simulink model "bpsk_simulink"  (Simulink 7.3)
settings: Solver=ode45  StartTime=0.0  StopTime=10.0  RelTol=1e-3
undefined symbols (not defined in the file or in its folder): get
libraries: commsink2 x4, commdigbbndpm3 x2, commfilt2 x2, dspsrcs4 x2, commchan3 x1, commrandsrc2 x1, commphrec2 x1, commrflib2 x1
settings Model: Creator=joneskoo  LastModifiedBy=joneskoo

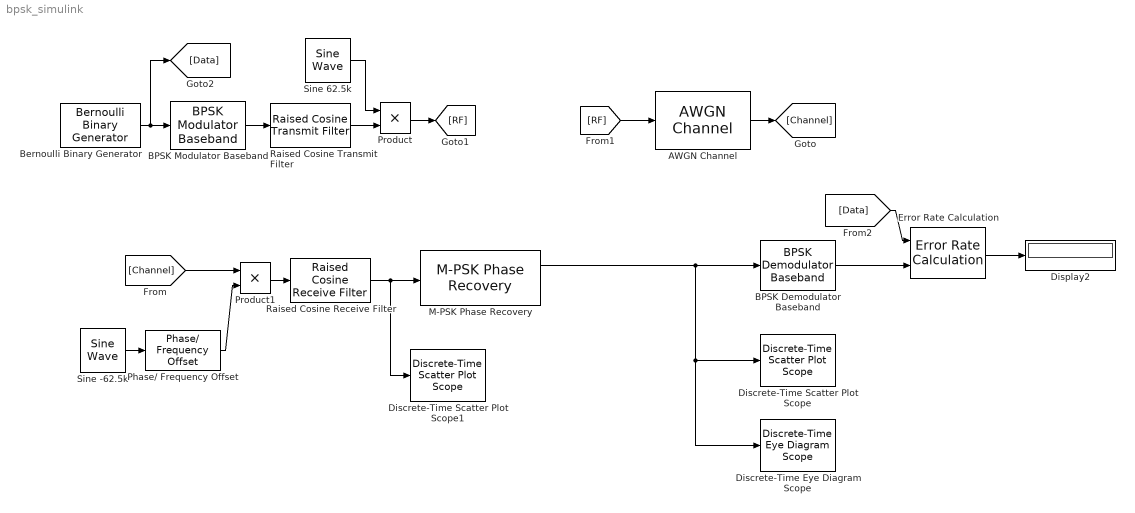
== system bpsk_simulink ==
  AWGN Channel : commchan3/AWGN Channel  SystemSampleTime=-1  seed=67  noiseMode="Signal to noise ratio  (SNR)"  EbNodB=40  EsNodB=10  SNRdB=15  bitsPerSym=1  Ps=1  Tsym=1  variance=1
  BPSK Demodulator Baseband : commdigbbndpm3/BPSK Demodulator Baseband  DialogController=commDDGCreate  DialogControllerArgs=DataTag0  Ph=0  DecType=Hard decision  VarSource=Dialog  Variance=1  outDtype=Inherit via internal rule  derotateFactorWordLen=16
  BPSK Modulator Baseband : commdigbbndpm3/BPSK Modulator Baseband  DialogController=commDDGCreate  DialogControllerArgs=DataTag1  SystemSampleTime=-1  Ph=0  outDtype=double  outWordLen=16  outUDDataType=sfix(16)  outFracLenMode=Best precision  outFracLen=15
  Bernoulli Binary Generator : commrandsrc2/Bernoulli Binary Generator  DialogController=commDDGCreate  DialogControllerArgs=DataTag2  SystemSampleTime=-1  P=0.5  seed=61  Ts=64/500000  frameBased=off  sampPerFrame=4  orient=off  outDataType=double
  Discrete-Time Eye Diagram Scope : commsink2/Discrete-Time Eye Diagram Scope  Tag=EyeDiagram  SystemSampleTime=-1  sampPerSymb=64  offsetEye=0  symbPerTrace=1  numTraces=40  numNewFrames=10  LineStyles=-  LineColors=b  dupPoints=on  fading=on  render=on  AxisGrid=on  yMin=-3.15  yMax=3.15  inphaseLabel=In-phase Amplitude  quadratureLabel=Quadrature Amplitude  openScopeAtSimStart=on  dispDiagram=In-phase and Quadrature  FrameNumber=off  FigPos=get(0,'defaultfigureposition');  figTitle=Eye Diagram  block_type_=eye  numLinesMax=8
  Discrete-Time Scatter Plot Scope : commsink2/Discrete-Time Scatter Plot Scope  Tag=ScatterPlot  SystemSampleTime=-1  sampPerSymb=64  offsetEye=0  numTraces=64  numNewFrames=2  LineMarkers=.  LineColors=b  fading=on  render=on  AxisGrid=on  xMin=-14.1164196040236  xMax=13.5450356467116  yMin=-13.1822502821127  yMax=14.4792049686224  inphaseLabel=In-phase Amplitude  quadratureLabel=Quadrature Amplitude  openScopeAtSimStart=on  FrameNumber=off  FigPos=get(0,'defaultfigureposition');  figTitle=Scatter Plot  numLinesMax=8  block_type_=scatter
  Discrete-Time Scatter Plot Scope1 : commsink2/Discrete-Time Scatter Plot Scope  Tag=ScatterPlot  SystemSampleTime=-1  sampPerSymb=64  offsetEye=0  numTraces=64  numNewFrames=2  LineMarkers=.  LineColors=b  fading=on  render=on  AxisGrid=on  xMin=-1.2305352029427  xMax=1.25246110954406  yMin=-1.24422807479241  yMax=1.23876823769434  inphaseLabel=In-phase Amplitude  quadratureLabel=Quadrature Amplitude  openScopeAtSimStart=on  FrameNumber=off  FigPos=get(0,'defaultfigureposition');  figTitle=Scatter Plot  numLinesMax=8  block_type_=scatter
  Display2 : Display
  Error Rate Calculation : commsink2/Error Rate Calculation  N=2  st_delay=0  cp_mode=Entire frame  subframe=[]  PMode=Port  WsName=ErrorVec  RsMode2=off  stop=off  numErr=100  maxBits=1e6
  M-PSK Phase Recovery : commphrec2/M-PSK Phase Recovery  SystemSampleTime=-1  M=2  intPeriod=10
  Phase/ Frequency Offset : commrflib2/Phase// Frequency Offset  phaseOffset=0  freqPort=off  freqOffset=0
  Product : Product  OutDataType=fixdt(1, 16)  OutScaling=2^0  RndMeth=Zero
  Product1 : Product  OutDataType=fixdt(1, 16)  OutScaling=2^0  RndMeth=Zero
  Raised Cosine Receive Filter : commfilt2/Raised Cosine Receive Filter  DialogController=dspDDGCreate  DialogControllerArgs=DataTag3  SystemSampleTime=-1  filtType=Square root  N=64  D=1  R=0.8  sampMode=Mute  saveAsFlag=0  framing=Maintain input frame size  rateMode=None  downFactor=64  downOffset=0  checkGain=Normalized  filterGain=1  checkCoeff=off  variableName=rcRxFilt  launchFVT=off  roundingMode=Floor  overflowMode=off
  Raised Cosine Transmit Filter : commfilt2/Raised Cosine Transmit Filter  DialogController=dspDDGCreate  DialogControllerArgs=DataTag4  SystemSampleTime=-1  filtType=Square root  D=1  R=0.8  sampMode=Mute  saveAsFlag=0  framing=Maintain input frame size  N=64  checkGain=Normalized  filterGain=10  checkCoeff=off  variableName=rcTxFilt  launchFVT=off  roundingMode=Floor  overflowMode=off
  Sine -62.5k : dspsrcs4/Sine Wave  Amplitude=1  Frequency=-62500  Phase=0  SampleMode=Discrete  OutComplex=Complex  CompMethod=Trigonometric fcn  TableSize=Speed  SampleTime=1/500000  SamplesPerFrame=1  dataType=double  wordLen=16  udDataType=sfix(16)  fracBitsMode=Best precision  numFracBits=15  ResetState=Restart at time zero
  Sine 62.5k : dspsrcs4/Sine Wave  Amplitude=1  Frequency=62500  Phase=0  SampleMode=Discrete  OutComplex=Complex  CompMethod=Trigonometric fcn  TableSize=Speed  SampleTime=1/500000  SamplesPerFrame=1  dataType=double  wordLen=16  udDataType=sfix(16)  fracBitsMode=Best precision  numFracBits=15  ResetState=Restart at time zero
  wires:
  Bernoulli Binary Generator/1 -> [Data], BPSK Modulator Baseband/1
  BPSK Modulator Baseband/1 -> Raised Cosine Transmit Filter/1
  Sine 62.5k/1 -> Product/1
  Product1/1 -> Raised Cosine Receive Filter/1
  Raised Cosine Receive Filter/1 -> M-PSK Phase Recovery/1, Discrete-Time Scatter Plot Scope1/1
  AWGN Channel/1 -> [Channel]
  Product/1 -> [RF]
  [RF] -> AWGN Channel/1
  [Channel] -> Product1/1
  Sine -62.5k/1 -> Phase/ Frequency Offset/1
  Phase/ Frequency Offset/1 -> Product1/2
  [Data] -> Error Rate Calculation/1
  BPSK Demodulator Baseband/1 -> Error Rate Calculation/2
  Error Rate Calculation/1 -> Display2/1
  M-PSK Phase Recovery/1 -> BPSK Demodulator Baseband/1, Discrete-Time Scatter Plot Scope/1, Discrete-Time Eye Diagram Scope/1
  Raised Cosine Transmit Filter/1 -> Product/2
